simulink model "voicecoil_meas"  (R2024a)
settings: Solver=ode3  StartTime=0.0  StopTime=0.3  FixedStep=Ts  RelTol=1e-4  AbsTol=1e-4
PostLoadFcn:
  | try
  | if isempty(which('ZHAWcbfcn'));
  | callback_fid07124=fopen('ZHAWcbfcn.m','w');
  | [~]=fprintf(callback_fid07124,'%s',get_param([bdroot,'/ Setup SLDRT'],'ClipboardFcn'));
  | [~]=fclose(callback_fid07124);
  | setpref('ZHAW_SLDRT_lib','cb_fcn',which('ZHAWcbfcn'))
  | clear callback_fid07124
  | end
  | catch
  | clear callback_fid07124
  | end
  | Ts=eval(get_param([bdroot,'/ Setup SLDRT'],'Ts'));
InitFcn:
  | Ts=eval(get_param([bdroot,'/ Setup SLDRT'],'Ts'));
values from neighbouring files (symbols this model uses):
  Kp = -(w0^2 - wcl^2)/(Ks*w0^2)    (= 1.5)    [voice_coil_ini.m]    (also in voicecoil.m = 9.79; voicecoilsim.m = 7.6346)
  Td = 0.005    [voicecoil.m]    (also in voicecoilsim.m = 0.0053)
  Ti = 0.49    [voicecoil.m]    (also in voicecoilsim.m = 0.2618)
undefined symbols (not defined in the file or in its folder): National_Instruments, PCIe
libraries: sldrtlib x3, cstblocks x1
(part 2 of 2)

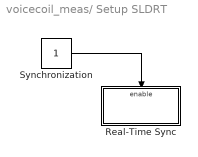
== system voicecoil_meas/ Setup SLDRT ==
  Real-Time Sync : Subsystem
  Synchronization : Constant
  wires:
  Synchronization/1 -> Real-Time Sync/Enable

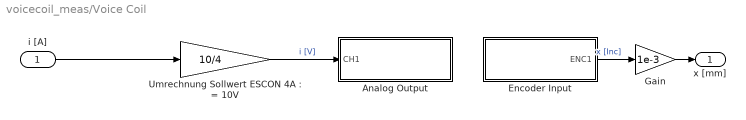
== system voicecoil_meas/Voice Coil ==
  i [A] : Inport
  Analog Output : Subsystem  mask(NI Analog Output){device=PCIe-6321, connect=Banana Terminal, ch1=on, ch2=off, ch3=off, ch4=off, Ts=Ts}
      mask prompts: device "NI Device Type:"; connect "Connector Box :"; Ts "Sample Time:"
      mask help:
      | DA Converter
      | +/- 10V
      mask init:
      | try ch_list = ZHAWcbfcn('get_ch_list'); end
      | try ZHAWcbfcn('BlockUpdate'); end
      settings: OpenFcn=try ZHAWcbfcn('openMask'); end
      settings: CopyFcn=|
      | try
      | ZHAWcbfcn('CopyIOblock')
      | end
      | set_param(gcb,'OpenFcn','try ZHAWcbfcn(''openMask''); end')
      mask TypeOptions device: PCI-6221 | PCI-6259 | PCIe-6259 | PCIe-6321 | PCIe-6363
      mask Callback device:
      | try ZHAWcbfcn('SetChannelNumber'); end
      | try ZHAWcbfcn('SetConnectorBox'); end
      mask TypeOptions connect: BNC Terminal | Banana Terminal | Screw Terminal
      mask Callback connect: try ZHAWcbfcn('SetConnectorBox'); end
      mask DialogControl DescGroupVar Prompt: NI Analog Output (R2024a)
      mask Display: disp('NI\nPCIe-6321')
  Encoder Input : Subsystem  mask(NI Encoder Input){device=PCIe-6321, connect=Banana Terminal, reset=off, ch1=on, ch2=off, ch3=off, ch4=off, Ts=Ts}
      mask prompts: device "NI Device Type:"; connect "Connector Box:"; reset "Reset at Index:"; ch1 "ENC1"; ch2 "ENC2"; ch3 "ENC3"; ch4 "ENC4"; Ts "Sample Time:"
      mask help:
      | Quadratur Encoder.
      | X4 Decoding.
      | Output is increments.
      mask init:
      | try ch_list = ZHAWcbfcn('get_ch_list'); end
      | try ZHAWcbfcn('BlockUpdate'); end
      settings: AttributesFormatString=Index Reset: %<reset>  OpenFcn=try ZHAWcbfcn('openMask'); end
      settings: CopyFcn=|
      | try
      | ZHAWcbfcn('CopyIOblock')
      | end
      | set_param(gcb,'OpenFcn','try ZHAWcbfcn(''openMask''); end')
      mask TypeOptions device: PCI-6221 | PCI-6259 | PCIe-6259 | PCIe-6321 | PCIe-6363
      mask Callback device: try ZHAWcbfcn('SetChannelNumber'); end
      mask TypeOptions connect: BNC Terminal | Banana Terminal | Screw Terminal
      mask Callback connect: try ZHAWcbfcn('SetConnectorBox'); end
      mask TypeOptions reset: on | off
      mask Callback reset: try ZHAWcbfcn('SetEncoderReset'); end
      mask DialogControl DescGroupVar Prompt: NI Encoder Input (R2024a)
      mask Display: disp('NI\nPCIe-6321')
  Gain : Gain  Gain=1e-3
  "Umrechnung Sollwert ESCON 4A : = 10V" : Gain  Gain=10/4
  x [mm] : Outport  VectorParamsAs1DForOutWhenUnconnected=off
  wires:
  Encoder Input/1(ENC1) -> Gain/1  "x [Inc]"
  "Umrechnung Sollwert ESCON 4A : = 10V"/1 -> Analog Output/1(CH1)  "i [V]"
  Gain/1 -> x [mm]/1
  i [A]/1 -> "Umrechnung Sollwert ESCON 4A : = 10V"/1

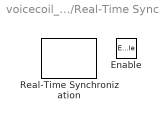
== system voicecoil_meas/ Setup SLDRT/Real-Time Sync ==
  Enable : EnablePort
  Real-Time Synchronization : sldrtlib/Real-Time Synchronization  SampleTime=Ts  MaxMissedTicks=inf  ShowMissedTicks=off  YieldWhenWaiting=off

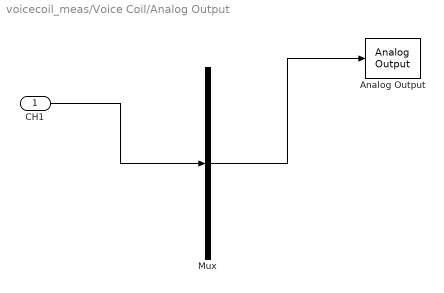
== system voicecoil_meas/Voice Coil/Analog Output ==
  CH1 : Inport
  Analog Output : sldrtlib/Analog Output  SampleTime=Ts  MaxMissedTicks=10  ShowMissedTicks=off  YieldWhenWaiting=off  DrvName=National_Instruments/PCIe-6321  DrvAddress=4294967295  DrvOptions="[1  0  0  2  2  2  2]"  Channels=ch_list  RangeMode=1  VoltRange=1  InitialValue=0  FinalValue=0
      settings: AttributesFormatString=National Instruments\nPCIe-6321 [auto]
  Mux : Mux  Inputs=1
  wires:
  Mux/1 -> Analog Output/1
  CH1/1 -> Mux/1

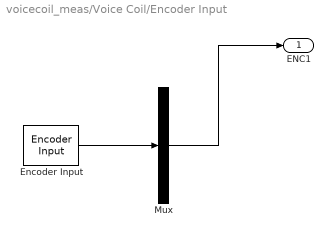
== system voicecoil_meas/Voice Coil/Encoder Input ==
  Encoder Input : sldrtlib/Encoder Input  SampleTime=Ts  MaxMissedTicks=10  ShowMissedTicks=off  YieldWhenWaiting=off  DrvName=National_Instruments/PCIe-6321  DrvAddress=4294967295  DrvOptions="[1  0  0  2  2  2  2]"  Channels=ch_list  QuadMode=3  IndexPulse=1  InputFilter=Inf  DataType=1
      settings: AttributesFormatString=National Instruments\nPCIe-6321 [auto]
  Mux : Demux  Outputs=1
  ENC1 : Outport  VectorParamsAs1DForOutWhenUnconnected=off
  wires:
  Encoder Input/1 -> Mux/1
  Mux/1 -> ENC1/1
